simulink model "Task9"  (R2024a)
settings: Solver=VariableStepAuto  StartTime=0.0  StopTime=10.0  RelTol=1e-3
settings Model: Creator=artemzmailov  LastModifiedBy=artemzmailov

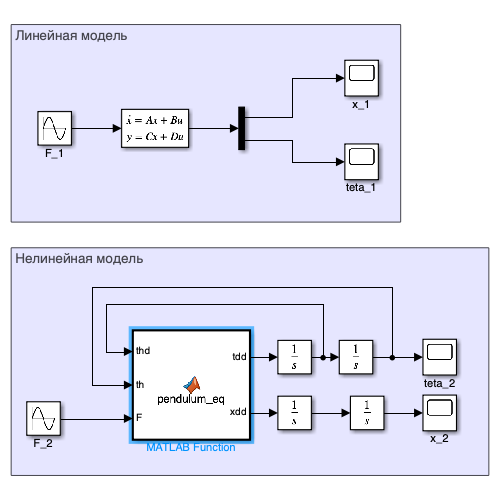
[thumbnail: Simulink's stored preview of the top-level diagram]
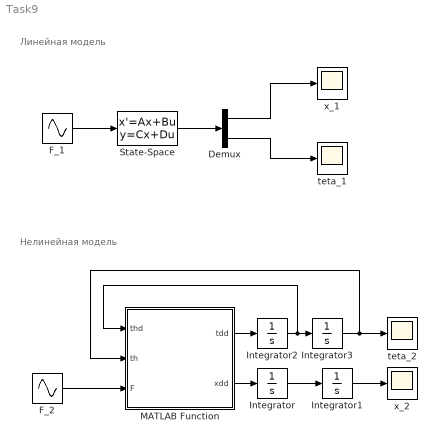
== system Task9 ==
  note: Нелинейная модель
  note: Линейная модель
  Demux : Demux  Outputs=2
  F_1 : Sin  Frequency=2  SampleTime=0
  F_2 : Sin  Frequency=2  SampleTime=0
  Integrator : Integrator  InitialCondition=0.5
  Integrator1 : Integrator
  Integrator2 : Integrator
  Integrator3 : Integrator
  MATLAB Function : MATLAB Function  TreatAsAtomicUnit=on
  State-Space : StateSpace  A=[0,1,0,0; 0,0,-2.4525,0; 0,0,0,1; 0,0,-32.7,0]  B=[0; 0.5; 0; -1.6667]  C=[1,0,0,0; 0,0,1,0]  D=[0;0]  InitialCondition=[0,0.5,0,0]
  teta_1 : Scope
  teta_2 : Scope
  x_1 : Scope
  x_2 : Scope
  wires:
  F_1/1 -> State-Space/1
  State-Space/1 -> Demux/1
  Demux/1 -> x_1/1
  Demux/2 -> teta_1/1
  F_2/1 -> MATLAB Function/3(F)
  MATLAB Function/2(xdd) -> Integrator/1
  Integrator/1 -> Integrator1/1
  Integrator2/1 -> MATLAB Function/1(thd), Integrator3/1
  MATLAB Function/1(tdd) -> Integrator2/1
  Integrator3/1 -> MATLAB Function/2(th), teta_2/1
  Integrator1/1 -> x_2/1

== matlab function Task9/MATLAB Function ==
  data: thd input; tdd output; xdd output; th input; F input
function [tdd, xdd] = pendulum_eq(thd, th, F)
    % th, thd — текущие состояния
    % Возвращает [xdd, tdd]
    
    % Решаем систему:
    % (M+m)*xdd + m*l*cos(th)*tdd = F + m*l*thd^2*sin(th)
    % cos(th)*xdd + l*tdd = -g*sin(th)
    M = 2;
    m = 0.5;
    l = 0.3;
    g = 9.81;

    A = [M+m, m*l*cos(th); cos(th), l];
    B = [F + m*l*thd^2*sin(th); -g*sin(th)];
    
    sol = A\B;
    xdd = sol(1);
    tdd = sol(2);
end
